simulink subsystem "cog_dyn_gci"  (R2022a)
settings: Solver=VariableStepAuto  StartTime=0.0  StopTime=10.0  RelTol=1e-3
settings Model: Creator=samuel  LastModifiedBy=samuel

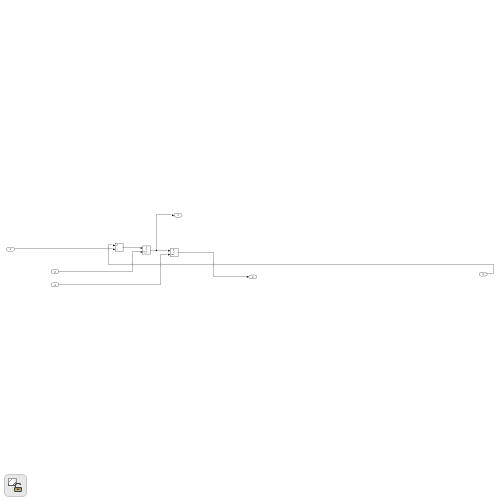
[thumbnail: Simulink's stored preview of the top-level diagram]
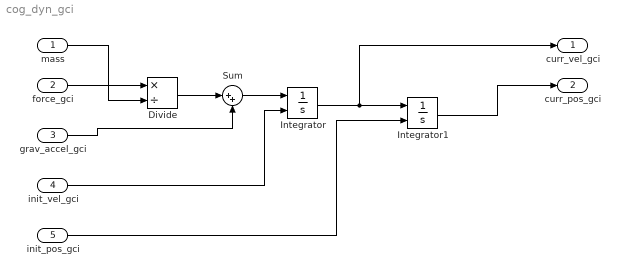
== system cog_dyn_gci ==
  mass : Inport
  force_gci : Inport  Port=2
  grav_accel_gci : Inport  Port=3
  init_vel_gci : Inport  Port=4
  init_pos_gci : Inport  Port=5
  Divide : Product  Inputs=*/
  Integrator : Integrator  InitialConditionSource=external
  Integrator1 : Integrator  InitialConditionSource=external
  Sum : Sum  Inputs=|++
  curr_vel_gci : Outport
  curr_pos_gci : Outport  Port=2
  wires:
  mass/1 -> Divide/2
  force_gci/1 -> Divide/1
  Integrator/1 -> curr_vel_gci/1, Integrator1/1
  init_pos_gci/1 -> Integrator1/2
  Integrator1/1 -> curr_pos_gci/1
  init_vel_gci/1 -> Integrator/2
  grav_accel_gci/1 -> Sum/2
  Divide/1 -> Sum/1
  Sum/1 -> Integrator/1
